simulink model "sm_car_Axle3"  (R2024a)
settings: Solver=ode23t  StartTime=0.0  StopTime=40  MaxStep=0.4  RelTol=1e-3  AbsTol=1e-3  EnableMultiTasking=on
PreLoadFcn:
  | % Due to usability issue in Repeating Sequence block
  | warning('off','Simulink:Masking:Invalid');
  | 
  | % Eliminate unnecessary warnings in inactive variants
  | % Warnings generated only if you click through inactive variant
  | warning('off','MATLAB:nonExistentField');
  | warning('off','Simulink:Parameters:BlkParamUndefined');
InitFcn:
  | warning('off','sm:sli:setup:compile:LocalSolverNotSupported')
  | sm_car_config_vehicle(bdroot);
  | sm_car_config_logging(bdroot);
  | 
  | % Check tire and vehicle model for correctness
  | Vehicle = sm_car_vehcfg_checkConfig(Vehicle);
  | sm_car_check_tire_model(bdroot);
StartFcn:
  | tic;
StopFcn:
  | Elapsed_Sim_Time = toc;
  | disp(['Elapsed Sim Time = ' num2str(Elapsed_Sim_Time)]);
undefined symbols (not defined in the file or in its folder): Axle1D, AxleIn, Camera, Control, Init, Init_Trailer, Maneuver, scenario, Scene, SimParams, Trailer, Visual, X, Y, Z
libraries: sm_lib x191, nesl_utility x84, fl_lib x43, simulink x15, Tire_Models x10, sdl_lib x8, Susp_DOF15 x5, sm_car_lib x3, sm_car_DSD_lib x3, drivingscenarioandsensors x1, sm_car_scene_crg_rough_road x1, sm_car_scene_double_lane_change x1
(part 4 of 11)

== system sm_car_Axle3/Vehicle/Vehicle ==
  In Bus Element2 : Inport  PortName=RdBus
  In Bus Element : Inport  Port=2  PortName=DrvBus
  In Bus Element3 : Inport  Port=2  PortName=DrvBus
  In Bus Element6 : Inport  Port=3  PortName=CtrlBus  Element=Brakes
  In Bus Element5 : Inport  Port=3  PortName=CtrlBus  Element=Chassis
  In Bus Element1 : Inport  Port=3  PortName=CtrlBus  Element=Power
  In Bus Element4 : Inport  Port=3  PortName=CtrlBus  Element=Driveline
  Body to World : Subsystem  mask(Body to World){Init=Init.Chassis, SpecifyPosTarget=on}
      mask prompts: Init "Initial Values"; SpecifyPosTarget "Specify Position Target"
      mask help: Models the connection between the vehicle body and world. Permits 6 degrees of freedom and sets the initial position, orientation, and speed of the vehicle body.
      mask init:
      | initial_aveh = [Init.aChassis.Value(3) Init.aChassis.Value(2) Init.aChassis.Value(1)];
      | rotmat_ypr = sm_car_yawpitchroll_to_rotmat(Init.aChassis.Value(3),Init.aChassis.Value(2),Init.aChassis.Value(1));
      | initial_vveh = rotmat_ypr*(Init.vChassis.Value)';
      | 
      | sptState = get_param(gcb,'SpecifyPosTarget');
      | 
      | set_param([gcb '/Body World Joint'],...
      |         'PxPositionTargetSpecify',sptState,...
      |         'PyPositionTargetSpecify',sptState,...
      |         'PzPositionTargetSpecify',sptState,...
      |         'SphPositionTargetSpecify',sptState,...
      |         'PxVelocityTargetSpecify',sptState,...
      |         'PyVelocityTargetSpecify',sptState,...
      |         'PzVelocityTargetSpecify',sptState...
      |         );
      mask Help: web('sm_car_doc_body_to_world.html')
  Brakes : Subsystem  Variant=on  VariantControlMode=label  VariantControl=Variant1  LabelModeActiveChoice=PedalAbstract_DiscDiscDisc  mask(Variants for Brake System){Brakes=Vehicle.Brakes, VariantLabel=Vehicle.Brakes.class.Value, InitTriggerDropdown=1}
      mask prompts: Brakes "Brake Parameters"; VariantLabel "Variant Label"; InitTriggerDropdown "Initialization Dropdown Trigger"
      mask help: Select option and provide parameters for brakes. Option is chosen by string provided in Variant Label. The parameters for the selected option is contained in Brakes data structure.
      mask init:
      | curblk = gcb;
      | 
      | % Set variant for this block 
      | set_param(curblk,'LabelModeActiveChoice',VariantLabel);
      | 
      | % Trigger Mask Initialization for 
      | % variant subsystems below this level
      | sm_car_lib_maskInitTrigger(curblk)
      settings: AttributesFormatString=%<ActiveVariant>
      mask TypeOptions InitTriggerDropdown: 0 | 1
      mask Display:
      | % Display same mask as active variant
      | blk = sm_car_lib_activeVariantBlock(gcb);
      | 
      | if(~isempty(blk))
      |     eval(get_param(blk, 'MaskDisplay'));
      | else
      |     disp(' ');
      | end
  Chassis : Subsystem  Tag=PublishSubsystem  VariantControl=Chassis  mask(Chassis){Chassis=Vehicle.Chassis, Init=Init, InitTriggerDropdown=1, mask_image_name=sm_car_vehicle_chassis_amandla3axle_IMAGE.png, veh_index=veh_index}
      mask prompts: Chassis "Vehicle Parameters"; Init "Initial Values"; InitTriggerDropdown "Initialization Trigger Dropdown"; mask_image_name "Mask Image (string)"; veh_index "Vehicle Index (for tires)"
      mask help: Models vehicle chassis, with suspension, body, tires, springs, and dampers.
      mask init:
      | curblk = gcb;
      | 
      | % Trigger Mask Initialization for 
      | % variant subsystems below this level
      | sm_car_lib_maskInitTrigger(curblk)
      mask Help: web('sm_car_doc_chassis.html')
      mask TypeOptions InitTriggerDropdown: 0 | 1
      mask Display:
      | % Get image from BodyGeometry.class
      | % (active choice for Body Geometry subsystem)
      | image('sm_car_chassis_cad_truck_amandla.png');
  Powertrain : Subsystem  mask{Powertrain=Vehicle.Powertrain, InitTriggerDropdown=1}
      mask prompts: Powertrain "Powertrain Parameters"; InitTriggerDropdown "Initialization Trigger Dropdown"
      mask init:
      | curblk = gcb;
      | 
      | % Trigger Mask Initialization for 
      | % variant subsystems below this level
      | sm_car_lib_maskInitTrigger(curblk)
      mask TypeOptions InitTriggerDropdown: 0 | 1
      mask Display: image('sm_car_vehicle_powertrain_IMAGE.png')
  C : PMIOPort  Side=Left
  W : PMIOPort  Port=2  Side=Left
  HitchR : PMIOPort  Port=3  Side=Left
  HitchF : PMIOPort  Port=4  Side=Right
  Out Bus Elemet5 : Outport  VectorParamsAs1DForOutWhenUnconnected=off  PortName=VehBus  Element=Chassis
  Out Bus Element : Outport  VectorParamsAs1DForOutWhenUnconnected=off  PortName=VehBus  Element=Brakes
  Out Bus Element1 : Outport  VectorParamsAs1DForOutWhenUnconnected=off  PortName=VehBus  Element=Driveline
  Out Bus Element2 : Outport  VectorParamsAs1DForOutWhenUnconnected=off  PortName=VehBus  Element=World
  Out Bus Element3 : Outport  VectorParamsAs1DForOutWhenUnconnected=off  PortName=VehBus  Element=Power
  wires:
  In Bus Element5/1 -> Chassis/3(CtrlBus)
  Brakes/1(" OutB") -> Out Bus Element/1
  Chassis/1(VehBus) -> [VehB], Out Bus Elemet5/1
  In Bus Element2/1 -> Chassis/2(RdBus)
  In Bus Element/1 -> Chassis/1(DrvBus)
  In Bus Element6/1 -> Brakes/2("CtrlBus ")
  Body to World/1(World) -> Out Bus Element2/1
  In Bus Element3/1 -> Brakes/1("DrvBus ")
  In Bus Element4/1 -> Powertrain/1(CtrlD)
  In Bus Element1/1 -> Powertrain/2(CtrlP)
  Powertrain/1(OutD) -> Out Bus Element1/1
  Powertrain/2(OutP) -> Out Bus Element3/1
  [VehB] -> Powertrain/3(VehB)
  connections:
  HitchR/RConn1 -- Chassis/LConn1
  Chassis/RConn4 -- Powertrain/RConn3
  Powertrain/RConn1 -- Chassis/RConn3
  Chassis/LConn3 -- Powertrain/LConn2
  Chassis/LConn2 -- Powertrain/LConn1
  Chassis/RConn5 -- Powertrain/RConn4 -- Brakes/RConn1
  Chassis/RConn6 -- Powertrain/RConn5 -- Brakes/RConn2
  Chassis/RConn7 -- Powertrain/RConn6 -- Brakes/RConn3
  Powertrain/LConn3 -- Chassis/LConn4 -- Brakes/LConn1
  Powertrain/LConn4 -- Chassis/LConn5 -- Brakes/LConn2
  Brakes/LConn3 -- Chassis/LConn6 -- Powertrain/LConn5
  C/RConn1 -- Chassis/RConn1 -- Body to World/LConn1
  Body to World/RConn1 -- W/RConn1
  HitchF/RConn1 -- Chassis/RConn2

== system sm_car_Axle3/Vehicle/Vehicle Constraint ==
  No Constraint : Subsystem  VariantControl=NoConstraint
  F : PMIOPort  Side=Right
  B : PMIOPort  Port=2  Side=Left

== system sm_car_Axle3/Visualization/Dashboard ==
  VehBus : Inport
  DrvBus : Inport  Port=2
  Accelerator Pedal : LinearGaugeBlock  LabelPosition=Hide  ScaleMax=1
  Brake Pedal : LinearGaugeBlock  ScaleMax=1
  Bus Selector : BusSelector  OutputSignals=Chassis.Body.CG.vx
  Bus Selector2 : BusSelector  OutputSignals=aSteerWheel,rAccelPedal,rBrakePedal
  Gain : Gain  Gain=180/pi
  Gain1 : Gain  Gain=3.6
  Speed (kph) : CustomWebBlock  LabelPosition=Hide  ShowInitialText=on  Configuration="{\"components\":[{\"name\":\"CircularScaleComponent\",\"settings\":{\"bounds\":{\"max\":100,\"min\":0,\"tickInterval\":\"auto\"},\"direction\":\"cw\",\"flipLimits\":0,\"innerRadius\":0.75,\"internalTickHeightScaleFactor\":1,\"labelColor\":[255,252,199],\"labelFont\":{\"font\":\"Arial\",\"fontSize\":12},\"labelRadius\":0.36,\"labelTransparency\":1,\"minorTickHeightScaleFactor\":0.2,\"needleImage\":{\"size\":[1890,567],\"src\":\"data:image\\/svg+xml;base64,PD94bWwgdmVyc2lvbj0iMS4wIiBlbmNvZGluZz0iVVRGLTgiIHN0YW5kYWxvbmU9Im5vIj8+CjxzdmcKICAgeG1sbnM6ZGM9Imh0dHA6Ly9wdXJsLm9yZy9kYy9lbGVtZW50cy8xLjEvIgogICB4bWxuczpjYz0iaHR0cDovL2NyZWF0aXZlY29tbW9ucy5vcmcvbnMjIgogICB4bWxuczpyZGY9Imh0dHA6Ly93d3cudzMub3JnLzE5OTkvMDIvMjItcmRmLXN5bnRheC1ucyMiCiAgIHhtbG5zOnN2Zz0iaHR0cDovL3d3dy53My5vcmcvMjAwMC9zdmciCiAgIHhtbG5zPSJodHRwOi8vd3d3LnczLm9yZy8yMDAwL3N2ZyIKICAgeG1sbnM6 ...(+4096 chars)\"},\"needleOffset\":[0.14,0],\"needleOrientation\":-45,\"needleRotation\":180,\"needleSize\":{\"height\":0.13,\"width\":0.41},\"outerRadius\":0.9,\"position\":[0.06486742424242424,0.05627705627705628,0.8917748917748918,0.8787878787878788],\"scaleAngle\":270,\"scaleAngleOffset\":135,\"scaleColors\":[],\"scaleColorsSize\":0.2,\"scalePosition\":[0,0,1,1],\"showLabels\":1,\"showMinorTicks\":1,\"showSpanLine\":1,\"showTicks\":1,\"tickColor\":[255,255,200],\"tickTransparency\":1,\"valueBarColor\":[0,114,189],\"valueBarPosition\":[0,0,1,1],\"valueBarSize\":0.2,\"valueBarTransparency\":1}},{\"name\":\"BackgroundImageComponent\",\"settings\":{\"image\":{\"size\":[500,500],\"src\":\"data:image\\/svg+xml;base64,PD94bWwgdmVyc2lvbj0iMS4wIiBlbmNvZGluZz0iVVRGLTgiIHN0YW5kYWxvbmU9Im5vIj8+CjxzdmcKICAgeG1sbnM6ZGM9Imh0dHA6Ly9wdXJsLm9yZy9kYy9lbGVtZW50cy8xLjEvIgogICB4bWxuczpjYz0iaHR0cDovL2NyZWF0aXZlY29tbW9ucy5vcmcvbnMjIgogICB4bWxuczpyZGY9Imh0dHA6Ly93d3cudzMub3JnLzE5OTkvMDIvMjItcmRmLXN5bnRheC1ucyMiCiAgIHhtbG5zOnN2Zz0iaHR0cDovL3d3dy53My5vcmcvMjAwMC9zdmciCiAgIHhtbG5zPSJodHRwOi8vd3d3LnczLm9yZy8yMDAwL3N2ZyIKICAgeG1sbnM6 ...(+9964 chars)\"},\"position\":[0,0,1,1],\"scaleMode\":\"0\"}},{\"name\":\"ForegroundImageComponent\",\"settings\":{\"image\":{\"size\":[0,0],\"src\":\"default\",\"srcOrientation\":[]},\"isForeground\":1,\"position\":[0,0,1,1],\"scaleMode\":\"0\"}}],\"legacySettings\":{\"BackgroundImage\":\"data:image\\/svg+xml;base64,PD94bWwgdmVyc2lvbj0iMS4wIiBlbmNvZGluZz0iVVRGLTgiIHN0YW5kYWxvbmU9Im5vIj8+CjwhLS0gR2VuZXJhdG9yOiBBZG9iZSBJbGx1c3RyYXRvciAxOS4yLjEsIFNWRyBFeHBvcnQgUGx1Zy1JbiAuIFNWRyBWZXJzaW9uOiA2LjAwIEJ1aWxkIDApICAtLT4KCjxzdmcKICAgeG1sbnM6ZGM9Imh0dHA6Ly9wdXJsLm9yZy9kYy9lbGVtZW50cy8xLjEvIgogICB4bWxuczpjYz0iaHR0cDovL2NyZWF0aXZlY29tbW9ucy5vcmcvbnMjIgogICB4bWxuczpyZGY9Imh0dHA6Ly93d3cudzMub3JnLzE5OTkvMDIvMjItcmRmLXN5bnRh ...(+9660 chars)\",\"CenterOffsetX\":\"0\",\"CenterOffsetY\":\"0\",\"GaugeArcColor\":\"#9ec0f7\",\"GaugeArcDefined\":\"true\",\"GaugeArcRadius\":\"0.1358563990074277\",\"GaugeArcRatio\":\"0.8333333333333\",\"GaugeArcRotation\":\"240.5385250290321\",\"GaugeArcStrokeWidth\":\"0.03972965542329953\",\"GaugeArcTransparency\":\"0\",\"GaugeMax\":\"150\",\"GaugeMin\":\"0\",\"GaugeTickColor\":\"#faf5c8\",\"GaugeTickTransparency\":\"1\",\"GaugeTickVisible\":\"true\",\"GaugeValue\":\"0\",\"NeedleHeight\":\"0.11602152693163792\",\"NeedleImage\":\"data:image\\/svg+xml;base64,PD94bWwgdmVyc2lvbj0iMS4wIiBlbmNvZGluZz0idXRmLTgiPz4KPCEtLSBHZW5lcmF0b3I6IEFkb2JlIElsbHVzdHJhdG9yIDE5LjIuMSwgU1ZHIEV4cG9ydCBQbHVnLUluIC4gU1ZHIFZlcnNpb246IDYuMDAgQnVpbGQgMCkgIC0tPgo8c3ZnIHZlcnNpb249IjEuMSIgeG1sbnM9Imh0dHA6Ly93d3cudzMub3JnLzIwMDAvc3ZnIiB4bWxuczp4bGluaz0iaHR0cDovL3d3dy53My5vcmcvMTk5OS94bGluayIgeD0iMHB4IiB5PSIwcHgiCgkgdmlld0JveD0iMCAwIDIwMCA1MCIgc3R5bGU9ImVuYWJsZS1iYWNrZ3JvdW5kOm5ldyAw ...(+9940 chars)\",\"NeedleInitialRotation\":\"-59.94322499147643\",\"NeedleWidth\":\"0.1911368983686954\",\"NeedleXPos\":\"0.3802298124325669\",\"NeedleYPos\":\"0.48117305677424654\",\"ScaleColorsJSON\":\"[]\",\"ValueArcColor\":\"#1759b0\",\"ValueArcTransparency\":\"1\"},\"settings\":{\"BindingType\":\"signal\",\"backgroundOffset\":0.14,\"backgroundOpacity\":1,\"fixedAspectRatio\":\"on\",\"showBackgroundColor\":0},\"type\":\"CircularGauge\"}"
  Steering Wheel Angle : SemiCircularGaugeBlock  LabelPosition=Hide  ScaleMin=-80  ScaleMax=80  TickInterval=20
  Terminator{,1..3} (4 alike) : Terminator
  wires:
  VehBus/1 -> Bus Selector/1
  DrvBus/1 -> Bus Selector2/1
  Bus Selector/1 -> Gain1/1  "<vx>"
  Gain/1 -> Terminator1/1  "aSteerWheel deg"
  Bus Selector2/3 -> Terminator3/1  "<rBrakePedal>"
  Bus Selector2/1 -> Gain/1  "<aSteerWheel>"
  Bus Selector2/2 -> Terminator2/1  "<rAccelPedal>"
  Gain1/1 -> Terminator/1  "Speed (kph)"

== system sm_car_Axle3/Visualization/Data for Unreal ==
  VehBus : Inport
  DrvBus : Inport  Port=2
  Bus Selector : BusSelector  OutputSignals=aSteerWheel
  Bus Selector1 : BusSelector  OutputSignals=World.x,World.y,World.z  OutputAsBus=on
  Bus Selector2 : BusSelector  OutputSignals=World.aRoll,World.aPitch,World.aYaw  OutputAsBus=on
  Bus Selector5 : BusSelector  OutputSignals=Chassis.WhlL1.n,Chassis.WhlR1.n,Chassis.WhlL2.n,Chassis.WhlR2.n
  Bus Selector6 : BusSelector  OutputSignals=Chassis.WhlL1.aCamber,Chassis.WhlR1.aCamber,Chassis.WhlL2.aCamber,Chassis.WhlR2.aCamber
  Mux : Mux
  Mux1 : Mux
  xyz : Outport  VectorParamsAs1DForOutWhenUnconnected=off
  rpy : Outport  Port=2  VectorParamsAs1DForOutWhenUnconnected=off
  ws : Outport  Port=3  VectorParamsAs1DForOutWhenUnconnected=off
  aCamber : Outport  Port=4  VectorParamsAs1DForOutWhenUnconnected=off
  aSteerWheel : Outport  Port=5  VectorParamsAs1DForOutWhenUnconnected=off
  wires:
  Bus Selector/1 -> aSteerWheel/1  "<aSteerWheel>"
  Bus Selector6/4 -> Mux1/4  "<aCamber>"
  Bus Selector6/3 -> Mux1/3  "<aCamber>"
  Bus Selector6/2 -> Mux1/2  "<aCamber>"
  Mux/1 -> ws/1  "ws"
  Bus Selector2/1 -> rpy/1  "rpy"
  Bus Selector6/1 -> Mux1/1  "<aCamber>"
  Bus Selector5/1 -> Mux/1  "<n>"
  Bus Selector5/2 -> Mux/2  "<n>"
  Bus Selector5/4 -> Mux/4  "<n>"
  DrvBus/1 -> Bus Selector/1
  VehBus/1 -> Bus Selector1/1, Bus Selector2/1, Bus Selector5/1, Bus Selector6/1
  Mux1/1 -> aCamber/1  "aCamber"
  Bus Selector1/1 -> xyz/1  "xyz"
  Bus Selector5/3 -> Mux/3  "<n>"

== system sm_car_Axle3/Visualization/Unreal ==
  "xyz " : Inport
  "rpy " : Inport  Port=2
  "ws " : Inport  Port=3
  "aCamber " : Inport  Port=4
  "aSteerWheel " : Inport  Port=5
  Animation Off : Subsystem  VariantControl=Off

== system sm_car_Axle3/Visualization/XY Plot ==
  "VehBus " : Inport
  "DrvBus " : Inport  Port=2
  XY Plot Off : Subsystem  VariantControl=Off

== system sm_car_Axle3/World/Mechanism Configuration ==
  Constant Gravity : Subsystem  VariantControl=ConstantGravity
  C : PMIOPort  Side=Right

== system sm_car_Axle3/World/Scene ==
  CRG Rough Road : sm_car_scene_crg_rough_road/CRG Rough Road  VariantControl=CRG_Rough_Road  geometry=Scene.CRG_Rough_Road.Geometry
  Double Lane Change : sm_car_scene_double_lane_change/Double Lane Change  VariantControl=Double_Lane_Change  road=Scene.Double_Lane_Change.Road  dashes=Scene.Double_Lane_Change.Dashes  cones=Scene.Double_Lane_Change.Cones
  Plane Grid : Subsystem  VariantControl=Plane_Grid  mask{plane=Scene.Plane_Grid.Plane, grid=Scene.Plane_Grid.Grid}
      mask prompts: plane "Ground Plane (structure)"; grid "Grid (structure)"
  Plane Grid1 : Subsystem  VariantControl=Plane Grid1  mask{plane=Scene.Plane_Grid.Plane, grid=Scene.Plane_Grid.Grid}
      mask prompts: plane "Ground Plane (structure)"; grid "Grid (structure)"
  W : PMIOPort  Side=Left
  Obs : Outport  VectorParamsAs1DForOutWhenUnconnected=off

== system sm_car_Axle3/Camera Frames/Dolly Camera/Off ==
  W : PMIOPort  Side=Left
  R : PMIOPort  Port=2  Side=Right
  connections:
  R/RConn1 -- W/RConn1

== system sm_car_Axle3/Controller/Default/Brake Control ==
  "rBrakePedal " : Inport
  "VehBus " : Inport  Port=2
  Pedal : Subsystem  VariantControl=Pedal
  " Brakes" : Outport  VectorParamsAs1DForOutWhenUnconnected=off
